simulink model "MATMPC_SIMULINK"  (R2019b)
settings: Solver=FixedStepAuto  StartTime=0.0  StopTime=1  RelTol=1e-3
undefined symbols (not defined in the file or in its folder): indata, opt, settings, Ts, x0
libraries: dspindex x1
settings Model: Creator=chen  LastModifiedBy=ichelikh
settings DataIOCC: ReturnWorkspaceOutputs=off
settings DebuggingCC: ArithmeticOperatorsInVariantConditions=warning
settings SFSimCC: SimUseLocalCustomCode=off  CustomCodeUndefinedFunction=UseInterfaceOnly
settings RTWCC: RTWUseLocalCustomCode=off  CheckMdlBeforeBuild=Error

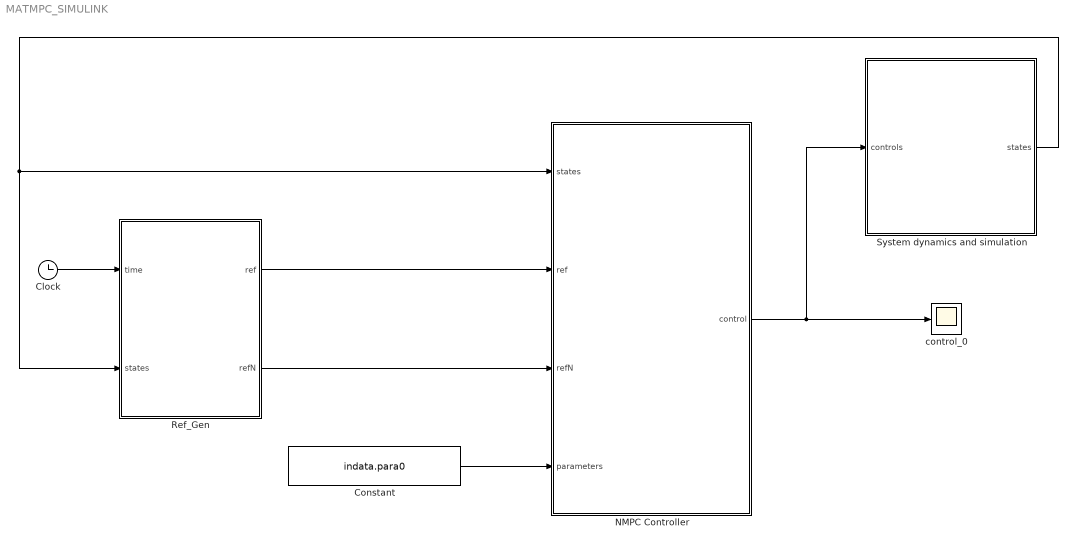
== system MATMPC_SIMULINK ==
  Clock : Clock
  Constant : Constant  Value=indata.para0
  NMPC Controller : Subsystem
  Ref_Gen : Subsystem
  System dynamics and simulation : Subsystem
  control_0 : Scope
  wires:
  NMPC Controller/1(control) -> System dynamics and simulation/1("controls "), control_0/1
  Ref_Gen/1(ref) -> NMPC Controller/2("ref ")
  Ref_Gen/2(refN) -> NMPC Controller/3("refN ")
  Constant/1 -> NMPC Controller/4(parameters)
  Clock/1 -> Ref_Gen/1(time)
  System dynamics and simulation/1(states) -> Ref_Gen/2("states "), NMPC Controller/1("states ")

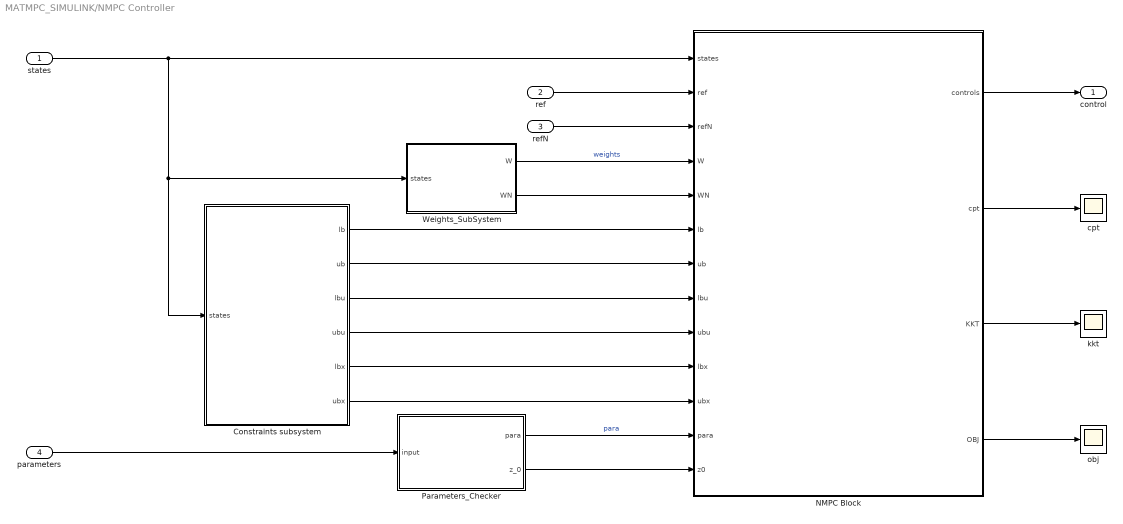
== system MATMPC_SIMULINK/NMPC Controller ==
  "states " : Inport
  "ref " : Inport  Port=2
  "refN " : Inport  Port=3
  parameters : Inport  Port=4
  Constraints subsystem : Subsystem
  "NMPC Block " : MATLAB Function  TreatAsAtomicUnit=on  SystemSampleTime=Ts
  Parameters_Checker : MATLAB Function  TreatAsAtomicUnit=on  SystemSampleTime=settings.Ts
  Weights_SubSystem : Subsystem
  cpt : Scope
  kkt : Scope
  obj : Scope
  control : Outport
  wires:
  "refN "/1 -> "NMPC Block "/3(refN)
  "NMPC Block "/4(OBJ) -> obj/1
  "NMPC Block "/3(KKT) -> kkt/1
  "NMPC Block "/2(cpt) -> cpt/1
  "ref "/1 -> "NMPC Block "/2(ref)
  "NMPC Block "/1(controls) -> control/1
  "states "/1 -> Constraints subsystem/1(states), Weights_SubSystem/1(states), "NMPC Block "/1(states)
  Weights_SubSystem/2(WN) -> "NMPC Block "/5(WN)
  Weights_SubSystem/1(W) -> "NMPC Block "/4(W)  "weights"
  Constraints subsystem/1(lb) -> "NMPC Block "/6(lb)
  Constraints subsystem/2(ub) -> "NMPC Block "/7(ub)
  Constraints subsystem/3(lbu) -> "NMPC Block "/8(lbu)
  Constraints subsystem/4(ubu) -> "NMPC Block "/9(ubu)
  Constraints subsystem/5(lbx) -> "NMPC Block "/10(lbx)
  Constraints subsystem/6(ubx) -> "NMPC Block "/11(ubx)
  Parameters_Checker/1(para) -> "NMPC Block "/12(para)  "para"
  parameters/1 -> Parameters_Checker/1(input)
  Parameters_Checker/2(z_0) -> "NMPC Block "/13(z0)

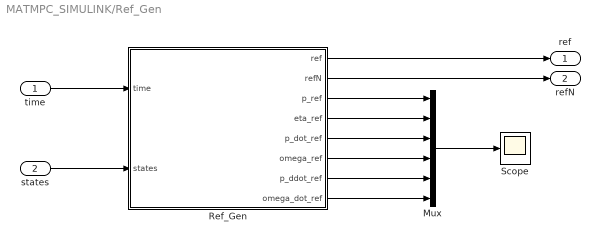
== system MATMPC_SIMULINK/Ref_Gen ==
  time : Inport
  "states " : Inport  Port=2
  Mux : Mux  Inputs=6
  Ref_Gen : MATLAB Function  TreatAsAtomicUnit=on
  Scope : Scope
  ref : Outport
  refN : Outport  Port=2
  wires:
  Ref_Gen/4(eta_ref) -> Mux/2
  Ref_Gen/3(p_ref) -> Mux/1
  Ref_Gen/8(omega_dot_ref) -> Mux/6
  Ref_Gen/2(refN) -> refN/1
  time/1 -> Ref_Gen/1(time)
  Ref_Gen/7(p_ddot_ref) -> Mux/5
  Ref_Gen/1(ref) -> ref/1
  Ref_Gen/5(p_dot_ref) -> Mux/3
  Ref_Gen/6(omega_ref) -> Mux/4
  Mux/1 -> Scope/1
  "states "/1 -> Ref_Gen/2(states)

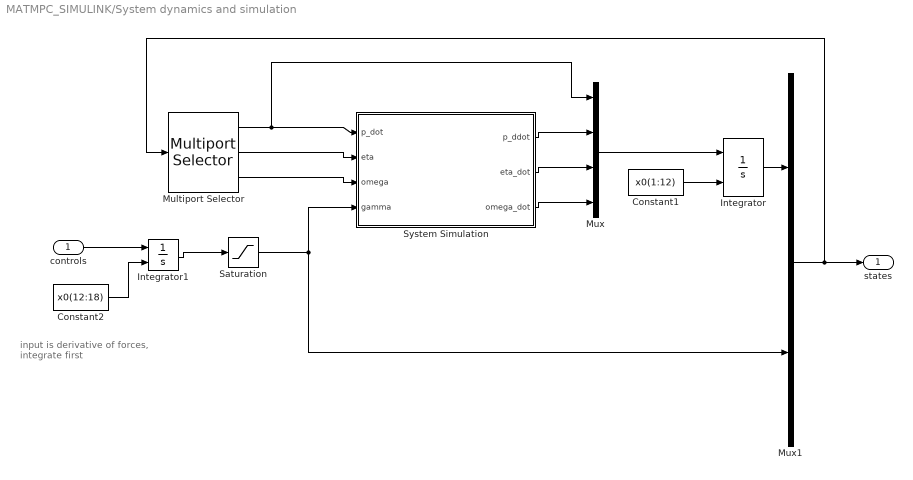
== system MATMPC_SIMULINK/System dynamics and simulation ==
  note: input is derivative of forces, integrate first
  "controls " : Inport
  Constant1 : Constant  Value=x0(1:12)
  Constant2 : Constant  Value=x0(12:18)
  Integrator : Integrator  InitialConditionSource=external  InitialCondition=x0
  Integrator1 : Integrator  InitialConditionSource=external
  Multiport Selector : dspindex/Multiport Selector  rowsOrCols=Rows  idxCellArray={ 4:6, 7:9, 10:12}  idxErrMode=Clip Index
  Mux : Mux
  Mux1 : Mux  Inputs=2
  Saturation : Saturate  UpperLimit=indata.constraints.f_max  LowerLimit=indata.constraints.f_min
  System Simulation : MATLAB Function  TreatAsAtomicUnit=on
  states : Outport
  wires:
  Integrator1/1 -> Saturation/1
  "controls "/1 -> Integrator1/1
  Saturation/1 -> Mux1/2, System Simulation/4(gamma)
  Multiport Selector/2 -> System Simulation/2(eta)
  Multiport Selector/3 -> System Simulation/3(omega)
  Constant1/1 -> Integrator/2
  Multiport Selector/1 -> Mux/1, System Simulation/1(p_dot)
  System Simulation/1(p_ddot) -> Mux/2
  System Simulation/2(eta_dot) -> Mux/3
  System Simulation/3(omega_dot) -> Mux/4
  Mux/1 -> Integrator/1
  Integrator/1 -> Mux1/1
  Mux1/1 -> states/1, Multiport Selector/1
  Constant2/1 -> Integrator1/2

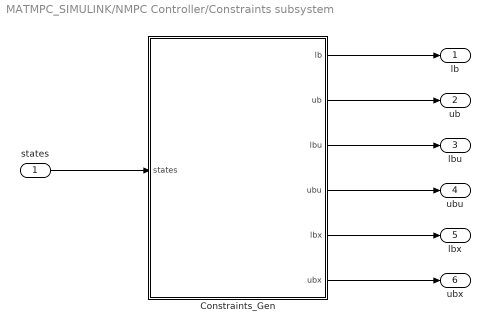
== system MATMPC_SIMULINK/NMPC Controller/Constraints subsystem ==
  states : Inport
  Constraints_Gen : MATLAB Function  TreatAsAtomicUnit=on  SystemSampleTime=settings.Ts
  lb : Outport  VectorParamsAs1DForOutWhenUnconnected=off
  ub : Outport  Port=2  VectorParamsAs1DForOutWhenUnconnected=off
  lbu : Outport  Port=3  VectorParamsAs1DForOutWhenUnconnected=off
  ubu : Outport  Port=4  VectorParamsAs1DForOutWhenUnconnected=off
  lbx : Outport  Port=5  VectorParamsAs1DForOutWhenUnconnected=off
  ubx : Outport  Port=6  VectorParamsAs1DForOutWhenUnconnected=off
  wires:
  states/1 -> Constraints_Gen/1(states)
  Constraints_Gen/5(lbx) -> lbx/1
  Constraints_Gen/3(lbu) -> lbu/1
  Constraints_Gen/6(ubx) -> ubx/1
  Constraints_Gen/1(lb) -> lb/1
  Constraints_Gen/2(ub) -> ub/1
  Constraints_Gen/4(ubu) -> ubu/1

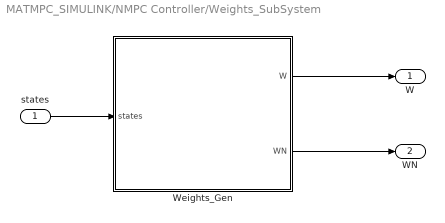
== system MATMPC_SIMULINK/NMPC Controller/Weights_SubSystem ==
  states : Inport
  Weights_Gen : MATLAB Function  TreatAsAtomicUnit=on  SystemSampleTime=settings.Ts
  W : Outport  VectorParamsAs1DForOutWhenUnconnected=off
  WN : Outport  Port=2
  wires:
  Weights_Gen/1(W) -> W/1
  states/1 -> Weights_Gen/1(states)
  Weights_Gen/2(WN) -> WN/1

== matlab function MATMPC_SIMULINK/System dynamics and simulation/System Simulation ==
  data: p_dot input size=3; eta input size=3; omega input size=3; gamma input size=nu; p_ddot output size=3; eta_dot output size=3; omega_dot output size=3; indata parameter
function [p_ddot,eta_dot,omega_dot] = Dynamic_System(p_dot, eta, omega, gamma, indata)

%% motion dynamics parameters definition
J = indata.model.J;
m = indata.model.m;
% Gravity [m/s^2]
% p     = [x; y; z];  Not needed: kept for consistency
% p_dot = [u, v, w];  Not needed: kept for consistency
% eta   = [phi; theta; psi];
% omega = eta_dot = [p; q; r];
% gamma = f = [f1; f2; f3; f4; f5; f6];

%% Extract variables

% ... from eta vector: needed to compute matrices R and T
phi = eta(1);
theta = eta(2);
psi = eta(3);

%% Initialize
g = 9.81; % gravity vector

O3 = zeros(3); % squared zero matrix of order 3
I3 = eye(3); % identity matrix of order 3
e3 = [0; 0; 1]; % z unit vector

% Generalised mass matrix
M = [m*I3 O3;
      O3  J ];

% Allocation matrix
G = [  -0.2449    0.2673   -0.2832    0.2496    0.6017   -0.5546
        0.4993   -0.4947   -0.4691    0.4971    0.0212   -0.0038
        0.7157    0.6958    0.6572    0.6714    0.7051    0.7304
       -0.0031    0.1762    0.1769   -0.0046   -0.1827   -0.1746
       -0.2100   -0.0996    0.0945    0.2112    0.1111   -0.1077
        0.1976   -0.1857    0.1864   -0.1945    0.1894   -0.1923    ];
 
% Rotation matrix from Euler Angles
r11 = cos(theta) * cos(psi);
r21 = cos(theta) * sin(psi);
r31 = -sin(theta);
r12 = sin(phi) * sin(theta) * cos(psi) - cos(phi) * sin(psi);
r22 = sin(phi) * sin(theta) * sin(psi) + cos(phi) * cos(psi);
r32 = sin(phi) * cos(theta);
r13 = cos(phi) * sin(theta) * cos(psi) + sin(phi) * sin(psi);
r23 = cos(phi) * sin(theta) * sin(psi) - sin(phi) * cos(psi);
r33 = cos(phi) * cos(theta);
R = [[r11 r21 r31].', [r12 r22 r32].', [r13 r23 r33].'];  

% Mapping matrix from eta_dot to omega
t11 = 1; t12 = 0;         t13 = -sin(theta);
t21 = 0; t22 = cos(phi);  t23 = sin(phi)*cos(theta);
t31 = 0; t32 = -sin(phi); t33 = cos(phi)*cos(theta);
T = [t11 t12 t13; t21 t22 t23; t31 t32 t33];

%% Dynamic equation of a floating-base rigid-body system

dyn_eq = M \ ([-m*g*e3; -cross(omega, J*omega)] + [R O3; O3 I3]*G*gamma);

%% Return output
% p_dot = p_dot; % unnecessary 
p_ddot = dyn_eq(1:3);
eta_dot = T \ omega;
omega_dot = dyn_eq(4:6);

return

== matlab function MATMPC_SIMULINK/NMPC Controller/NMPC Block  ==
  settings: updateMethod=DISCRETE
  data: states input size=nx; opt parameter; ref input size=[ny N]; refN input size=nyN; controls output size=[nu 1]; cpt output size=1; KKT output; OBJ output; W input; WN input; lb input; ub input; lbu input; ubu input; lbx input; ubx input; settings parameter; para input; z0 input
function [controls, cpt, KKT, OBJ] = NMPC_BLOCK(states, opt, ref, refN, W, WN, lb, ub, lbu, ubu, lbx, ubx, settings, para, z0)

%% everything should has a fixed size
coder.extrinsic('mpc_nmpcsolver_simulink');  
coder.extrinsic('InitData');  
coder.extrinsic('InitMemory');  
coder.extrinsic('evalin');
coder.extrinsic('assignin');

%%

persistent x u z lambda mu mu_x mu_u;
persistent input mem;

if isempty(input)  
    
    nx = settings.nx;        % No. of differential states
    nu = settings.nu;        % No. of controls
    nz = settings.nz;        % No. of algebraic states
    ny = settings.ny;        % No. of outputs (references)    
    nyN= settings.nyN;       % No. of outputs at terminal stage 
    np = settings.np;        % No. of parameters (on-line data)
    nc = settings.nc;        % No. of constraints
    ncN = settings.ncN;      % No. of constraints at terminal stage
    nbu = settings.nbu;      % No. of control bounds
    nbx = settings.nbx;      % No. of state bounds
    nbu_idx = settings.nbu_idx; % Index of control bounds
    nbx_idx = settings.nbx_idx; % Index of state bounds
    N = settings.N;
    N2 = settings.N2;
    r = settings.r;
        
    input.x0=states;
    
    x=repmat(states,1,N+1);
    input.x=x;
    
    u=zeros(nu,N);
    input.u=u;
    
    z=repmat(z0,1,N);
    input.z=z;
    
    lambda = zeros(nx,N+1);
    input.lambda= lambda;
    
    if N*nc+ncN > 0
        mu = zeros(N*nc+ncN,1);
    else
        mu = 0;
    end
    input.mu= mu;
    
    mu_u = zeros(N*nu,1);
    input.mu_u= mu_u;
    
    if N*nbx > 0
        mu_x = zeros(N*nbx,1);
    else
        mu_x = 0;
    end
    input.mu_x = mu_x;
    
    input.W=W;
    input.WN=WN;
    input.od = para;
    
    input.lb = lb;
    input.ub = ub;
    input.lbx = lbx;
    input.ubx = ubx;
    input.lbu = lbu;
    input.ubu = ubu;
      
    input.y = ref;
    input.yN = refN;
    
    mem = InitMemory(settings, opt, input);
        
else

    input.x=x; 
    input.u=u;
    input.z=z;
    input.lambda=lambda;   
    input.mu=mu;
    input.mu_x=mu_x;
    input.mu_u=mu_u;
    
end

%%
cpt = 0;
KKT = 0;
OBJ = 0;
input.x0 = states;
[input,mem,cpt,KKT,OBJ] = mpc_nmpcsolver_simulink(input, settings, mem, opt);
controls = input.u(:,1);

%% shifting
switch opt.shifting
    case 'yes'
        x=[input.x(:,2:end),input.x(:,end)];  
        u=[input.u(:,2:end),input.u(:,end)]; 
        z=[input.z(:,2:end),input.z(:,end)]; 
        lambda=[input.lambda(:,2:end),input.lambda(:,end)];
        if (settings.N*settings.nc+settings.ncN) >0
            mu(1:end-settings.ncN+1)=input.mu(settings.nc+1:settings.N*settings.nc+settings.ncN,1);
            mu(settings.N*settings.nc+1:end)=input.mu(settings.N*settings.nc+settings.ncN-settings.nc+1:settings.N*settings.nc+settings.ncN,1);
        else
            mu=0;
        end
        mu_x=[input.mu_x(2:end,1);input.mu_x(end,1)];
        mu_u=[input.mu_u(2:end,1);input.mu_u(end,1)];
   case 'no'
        x=input.x;
        u=input.u;
        z=input.z;
        lambda=input.lambda;
        mu=input.mu;
        mu_x=input.mu_x;
        mu_u=input.mu_u;
end

return

== matlab function MATMPC_SIMULINK/Ref_Gen/Ref_Gen ==
  data: ref output; settings parameter; refN output; time input; states input size=nx; p_ref output; eta_ref output; p_dot_ref output; omega_ref output; p_ddot_ref output; omega_dot_ref output; indata parameter
function [ref, refN, p_ref, eta_ref, p_dot_ref, omega_ref, p_ddot_ref, omega_dot_ref] = Reference_Gen(settings, time, states, indata)

persistent j motion t_start desired_WP tau W_p_B WPs;
            
%% Import variables
% ... from struct "settings"
N = settings.N;
ny = settings.ny;
nyN = settings.nyN;
nu_v = settings.nu_v;
nu_lambda = settings.nu_lambda;
Ts_st = settings.Ts_st;

% ... from vector "data"
x0 = indata.x0;

%% Initialize vectors

curr_pos = zeros(3, 1);
ref = zeros(ny, N);
refN = zeros(nyN, 1);

REF = zeros(ny, (N + 1));

p_ref = zeros(3, 1); 
eta_ref = zeros(3, 1); 
p_dot_ref = zeros(3, 1); 
omega_ref = zeros(3, 1); 
p_ddot_ref = zeros(3, 1); 
omega_dot_ref = zeros(3, 1);

%% Take current state
curr_pos(1) = states(1); % At the beginning states is equal to x0 (see Initialization_Simulink.m)
curr_pos(2) = states(2);
curr_pos(3) = states(3); 

%% Initialize default values for reference trajectory
% Some may be overwritten in next section

% Default values for desired position
x = 0; 
y = 0; 
z = 0;
% Default values for desired linear velocity
x_dot = 0; 
y_dot = 0; 
z_dot = 0;
% Default values for desired acceleration
x_ddot = 0; 
y_ddot = 0; 
z_ddot = 0;
% Default values for desired attitude
roll = 0; 
pitch = 0;             
yaw = 0; 
% Default values for desired angular velocity
omega_x = 0; 
omega_y = 0; 
omega_z = 0;
% Default values for desired angular acceleration
omega_dot_x = 0;
omega_dot_y = 0;
omega_dot_z = 0;
    
%% Generate reference trajectory
for i = 1: N+1
        
  % ........................ Sequence of waypoints ......................
  p_t0 = indata.x0(1:3); % starting position --- p(t=t0)
  h_safe = 0; % safety-height offset
  av_speeds = indata.wps.vel; % import speeds steps
  n_wps = indata.wps.num; % import number of waypoints
  if isempty(desired_WP)
      j = 1; 
      WPs = indata.wps.pos; % load sequence of waypoints
      desired_WP = WPs(:,j); % set as desired waypoint the current one
      % initialize body position in World frame (where drone 
      % should be at current time t)
      W_p_B = p_t0 + [0; 0; h_safe]; 
      t_start = indata.wps.t_start; % import time instant in which motion should start
      tau = 1;
      motion = 0;
  end
  if (time > t_start) && ~motion && j < n_wps
      desired_WP = WPs(:, j+1); % set as desired waypoint the next one
      distances = sqrt((desired_WP - WPs(:,j)).^2); % compute distance to next waypoint
      % compute time needed to reach next waypoint using 
      % corresponding constant speed step
      tau = norm(distances)/ 4.5 / av_speeds(j); 
      if tau > 0.001 % if next waypoint if far enough
          motion = 1; % trigger motion
      end
  end
  if motion % if motion has been triggered
      t = (time - t_start) / tau;
      % compute position where drone should be at current time t,
      % through a 2nd-order system response to motion step
      W_p_B = WPs(:,j) + (desired_WP - WPs(:,j)) .* (1 - exp(-t) - t*exp(-t)); 
      if norm(W_p_B - desired_WP) < 0.01 % if next waypoint has been reached
          disp('drone waypoint reached');
          disp(j+1);
          j = j+1; % point to next waypoint
          motion = 0; % reset motion trigger
          t_start = time + indata.wps.t_rest; % wait rest time before start next motion step
      end
  end
  % set as desired coordinates the position where drone should be
  % at current time t
  x = W_p_B(1); 
  y = W_p_B(2);
  z = W_p_B(3);
  % set desired yaw
  yaw = x0(9);


% Return desired reference trajectory of first shooting point for
% plotting purposes
if i == 1
    p_ref = [x y z]';
    p_dot_ref = [x_dot y_dot z_dot]';
    p_ddot_ref = [x_ddot y_ddot z_ddot]';

    eta_ref = [roll pitch yaw]';
    omega_ref = [omega_x omega_y omega_z]';
    omega_dot_ref = [omega_dot_x omega_dot_y omega_dot_z]';
end

% Reference over the time window for NMPC
REF(:, i) = [ x y z ...     % p
              roll pitch yaw ...    % eta
              x_dot y_dot z_dot ...     % p_dot
              omega_x omega_y omega_z ...   % omega
              x_ddot y_ddot z_ddot ...  % p_ddot
              omega_dot_x omega_dot_y omega_dot_z ...  % omega_dot
              0*ones(nu_v,1)' ...   % alpha_dot
              0*ones(nu_lambda,1)']'; %lambda_dot

end

%% Return output
ref = REF(:, 1:N);
refN = REF(1:end-nu_v-nu_lambda, N+1);

== matlab function MATMPC_SIMULINK/NMPC Controller/Constraints subsystem/Constraints_Gen ==
  settings: sampleTime=sim_time_step
  data: lb output size=settings.size_b; settings parameter; indata parameter; states input size=settings.nx; ub output size=settings.size_b; lbu output size=settings.size_bu; ubu output size=settings.size_bu; lbx output size=settings.size_bx; ubx output size=settings.size_bx
function [lb, ub, lbu, ubu, lbx, ubx]  = Constraints_Gen(settings, indata, states)

%% Importing 
% ... from  parameter `settings`
nu = settings.nu;
nu_lambda = settings.nu_lambda;
nu_v = settings.nu_v;
nbu = settings.nbu;
nbu_idx = settings.nbu_idx;
N = settings.N;

% ... from parameter `data`
c_f = indata.model.c_f;
omega_bar = indata.constraints.omega_bar;
dot_omega_bar_max = indata.constraints.dot_omega_bar_max;
dot_omega_bar_min = indata.constraints.dot_omega_bar_min;
coeff_angular_acc = indata.constraints.coeff_angular_acc;
coeff_angular_dec = indata.constraints.coeff_angular_dec;
%
dot_alpha_min = indata.constraints.dot_alpha_min;
dot_alpha_max = indata.constraints.dot_alpha_max;

% ... from input `states`
% State-dependent constraints
F = zeros(0,1);
for k = 0:nu-1
    F = [F;states(13+k)];
end
% f1 = states(13);
% f2 = states(14);
% f3 = states(15);
% f4 = states(16);
% f5 = states(17);
% f6 = states(18);

%% Variables definition

% vector F
% F = [f1; f2; f3; f4; f5; f6];

% Define the bounds of Delta U from equation:
%   dot_f(t) = 2 * kf * omega_i(t) * dot_omega_i(t),
%   where i is the i-th propeller 

%% Upper and lower bounds for general constraints 
% Dimensions of lb_g and ub_g should be equal to nc.
lb_g = [];
ub_g = [];

% Dimensions of lb_gN and ub_gN should be equal to ncN.
lb_gN = [];
ub_gN = [];

lb_g_rep = repmat(lb_g, N, 1);
ub_g_rep = repmat(ub_g, N, 1);

lb_temp = [lb_g_rep; lb_gN];
ub_temp = [ub_g_rep; ub_gN];

if isempty(lb_temp | ub_temp)
    
    lb = 0;
    ub = 0;

else
    
    lb = lb_temp;
    ub = ub_temp;
    
end

%% Lower and upper bounds for input 
% Dimensions of lb_u and ub_u should be equal to nbu.
lb_u = zeros(nbu, 1);
ub_u = zeros(nbu, 1);

% Propeller upper and lower bounds computation
% The bounds depend on current state of TiltHex. 
% This computation is repeated for each propeller
dot_omega_temp_acc = zeros(nu_lambda, 1);
dot_omega_temp_dec = zeros(nu_lambda, 1);

for i = 1:nu_lambda
% At each value inside omega_bar corresponds an upper and lower bound of dot_omega_bar,
% taken rispectively inside dot_omega_bar_max and dot_omega_bar_min.
% First it is mandatory to understand in which interval is the force provided
% by the i-th propeller; omega_bar values are translated into force
% quantities by F = k_f*omega^2 relationship, then i-th propeller's force is 
% compared to those value in order to understand in which interval the i-th 
% propeller is working. Then, once found the interval, linear interpolation 
% is used to adjust upper and lower bounds of extremity points of that
% interval to the actual in-between point.
        
        % If less force is requested w.r.t. the first upper and lower
        % bounds, then use first elements of omega_bar_min and _max
        % AND ALSO (update Davide & Youssef 01/06/2021) set the lower and
        % upper limits for the input equal to the same limits of the first
        % (smaller) spinning velocity setpoint. 
        % This is done to avoid the if a propeller is spinnijg with zero
        % velocity also his bounds of acceleration are set to zero; we
        % don't want this. Therefore, a minimum acceleration/deceleration
        % is always guaranteed.
        f_first_setpoint = c_f(i) * omega_bar(1)^2;
        if (abs(F(i)) <= f_first_setpoint)
            dot_omega_temp_acc(i) = dot_omega_bar_max(1);
            dot_omega_temp_dec(i) = dot_omega_bar_min(1);
            ub_u(i) = 2 * sqrt(f_first_setpoint * c_f(i)) * dot_omega_bar_max(1);
            lb_u(i) = 2 * sqrt(f_first_setpoint * c_f(i)) * dot_omega_bar_min(1);
        
        % Otherwise you need to interpolate, depending at which omega the
        % i-th propeller is spinning. 
        elseif (abs(F(i)) > c_f(i) * omega_bar(1)^2 && abs(F(i)) <= c_f(i) * omega_bar(2)^2)
            dot_omega_temp_acc(i) = (coeff_angular_acc(1) * (sqrt(abs(F(i)) / c_f(i)) - omega_bar(2)) + dot_omega_bar_max(2));
            dot_omega_temp_dec(i) = (coeff_angular_dec(1) * (sqrt(abs(F(i)) / c_f(i)) - omega_bar(2)) + dot_omega_bar_min(2));
            ub_u(i)= 2 * sqrt(abs(F(i)) * c_f(i)) * dot_omega_temp_acc(i);
            lb_u(i)= 2 * sqrt(abs(F(i)) * c_f(i)) * dot_omega_temp_dec(i);
            
        elseif (abs(F(i)) > c_f(i) * omega_bar(2)^2 && abs(F(i)) <= c_f(i) * omega_bar(3)^2)
            dot_omega_temp_acc(i) = (coeff_angular_acc(2) * (sqrt(abs(F(i)) / c_f(i)) - omega_bar(3)) + dot_omega_bar_max(3));
            dot_omega_temp_dec(i) = (coeff_angular_dec(2) * (sqrt(abs(F(i)) / c_f(i)) - omega_bar(3)) + dot_omega_bar_min(3));
            ub_u(i) = 2 * sqrt(abs(F(i)) * c_f(i)) * dot_omega_temp_acc(i);
            lb_u(i) = 2 * sqrt(abs(F(i)) * c_f(i)) * dot_omega_temp_dec(i);
        
        elseif (abs(F(i)) > c_f(i) * omega_bar(3)^2 && abs(F(i)) <= c_f(i) * omega_bar(4)^2)
            dot_omega_temp_acc(i) = (coeff_angular_acc(3) * (sqrt(abs(F(i)) / c_f(i)) - omega_bar(4)) + dot_omega_bar_max(4));
            dot_omega_temp_dec(i) = (coeff_angular_dec(3) * (sqrt(abs(F(i)) / c_f(i)) - omega_bar(4)) + dot_omega_bar_min(4));
            ub_u(i) = 2 * sqrt(abs(F(i)) * c_f(i)) * dot_omega_temp_acc(i);
            lb_u(i) = 2 * sqrt(abs(F(i)) * c_f(i)) * dot_omega_temp_dec(i);
        
        elseif (abs(F(i)) > c_f(i) * omega_bar(4)^2 && abs(F(i)) <= c_f(i) * omega_bar(5)^2)
            dot_omega_temp_acc(i) = (coeff_angular_acc(4) * (sqrt(abs(F(i)) / c_f(i)) - omega_bar(5)) + dot_omega_bar_max(5));
            dot_omega_temp_dec(i) = (coeff_angular_dec(4) * (sqrt(abs(F(i)) / c_f(i)) - omega_bar(5)) + dot_omega_bar_min(5));
            ub_u(i)= 2 * sqrt(abs(F(i)) * c_f(i)) * dot_omega_temp_acc(i);
            lb_u(i)= 2 * sqrt(abs(F(i)) * c_f(i)) * dot_omega_temp_dec(i);
        
        elseif (abs(F(i)) > c_f(i) * omega_bar(5)^2 && abs(F(i)) <= c_f(i) * omega_bar(6)^2)
            dot_omega_temp_acc(i) = (coeff_angular_acc(5) * (sqrt(abs(F(i)) / c_f(i)) - omega_bar(6)) + dot_omega_bar_max(6));
            dot_omega_temp_dec(i) = (coeff_angular_dec(5) * (sqrt(abs(F(i)) / c_f(i)) - omega_bar(6)) + dot_omega_bar_min(6));
            ub_u(i) = 2 * sqrt(abs(F(i)) * c_f(i)) * dot_omega_temp_acc(i);
            lb_u(i) = 2 * sqrt(abs(F(i)) * c_f(i)) * dot_omega_temp_dec(i);
        
        elseif (abs(F(i)) > c_f(i) * omega_bar(6)^2)
            dot_omega_temp_acc(i) = (coeff_angular_acc(6) * (sqrt(abs(F(i)) / c_f(i)) - omega_bar(7)) + dot_omega_bar_max(7));
            dot_omega_temp_dec(i) = (coeff_angular_dec(6) * (sqrt(abs(F(i)) / c_f(i)) - omega_bar(7)) + dot_omega_bar_min(7));
            ub_u(i) = 2 * sqrt(abs(F(i)) * c_f(i)) * dot_omega_temp_acc(i);
            lb_u(i) = 2 * sqrt(abs(F(i)) * c_f(i)) * dot_omega_temp_dec(i);
        end
end

%
for i = nu_lambda+1:nu_lambda+nu_v
    ub_u(i) = dot_alpha_max;
    lb_u(i) = dot_alpha_min;   
end
%

lbu_temp = -inf(nu, 1);
ubu_temp = inf(nu, 1);

for i = 1:nbu
    lbu_temp(nbu_idx(i)) = lb_u(i);
    ubu_temp(nbu_idx(i)) = ub_u(i);
end

lbu = repmat(lbu_temp, 1, N);
ubu = repmat(ubu_temp, 1, N);

%% Lower and upper bounds for state 
lb_x = indata.constraints.lbx;
ub_x = indata.constraints.ubx;

if isempty(lb_x | ub_x)    
    lbx = zeros(1, N);
    ubx = zeros(1, N);
else
    lbx = repmat(lb_x, 1, N);
    ubx = repmat(ub_x, 1, N);
end

end

== matlab function MATMPC_SIMULINK/NMPC Controller/Parameters_Checker ==
  data: para output size=settings.size_od; settings parameter; input input; z_0 output
function [para, z_0]  = Parameters_Checker(settings, input)
% PARA_GENERATOR Prepares para matrix for NMPC solver. 
%
% Para is a matrix containing all the params values over all shooting
% points. Each column j is a vector containing params values for the j-th
% shooting point. Therefore the para matrix must have the number of rows
% equal to the number of params and number of columns equal to N+1, where N
% is the number of shooting points.
%
%   para PARA_GENERATOR(input, settings)
%     
%     Inputs:
%     ---------------------------------------------------------------------
%       - input: struct containing all params. Each field is a different
%                param
%
%       - settings: struct containing data related to the settings used in
%                   the simulation
%           -> Ts: sampling time [s] (i.e. time at which the controller
%                  works)
%           -> Ts_st: shooting interval [s], i.e. temporal distance between 
%                     one shooting point and the next one
%           -> s: number of integration steps per interval
%           -> nx: no. of states
%           -> nu: no. of controls
%           -> ny: no. of outputs (references)    
%           -> nyN: no. of outputs at terminal stage 
%           -> np: no. of parameters (on-line data)
%           -> nc: no. of constraints
%           -> ncN: no. of constraints at terminal stage
%           -> nbu: no. of control bounds
%           -> nbx: no. of state bounds
%           -> nbu_idx: index of control bounds
%           -> nbx_idx: index of state bounds
%           -> N: no. of shooting points
%           -> N2: no. of partial condensing blocks 
%           -> r: no. of input move blocks
%
%     Outputs:
%     ---------------------------------------------------------------------
%       - para: matrix containing all the params values over all shooting
%               points. Each column j is a vector containing params values 
%               for the j-th shooting point. Its dimension is
%               [no_of_params, N+1], where N is the number of shooting
%               points

    %% Extracting variables from settings struct
    
    % Number of shooting points
    N = settings.N;
    np = settings.np;
    nz = settings.nz;
    %% Arraging params in para vector
    % para must be a matrix, where each column j is the vector of params of
    % the j-th shooting point
    
    if np > 0
        input_rows = size(input, 1);
        input_columns = size(input, 2);
        if input_rows == np && input_columns == N+1
            para = input;
        else
            error('NMPC para vector has invalid size!');
        end
    else
        para = zeros(1, N+1); % see settings.size_od
    end
    z_0 = settings.z0;
     % faire un bloc espace algebrique 
    % Sice at the beginning of the NMPC solver this param is constant over
    % all shooting points, replicate it over n+1 column
%     para = repmat(params, 1, N+1); % dimension = [n_of_params, N+1], where N is the number of shooting points
end

== matlab function MATMPC_SIMULINK/NMPC Controller/Weights_SubSystem/Weights_Gen ==
  settings: sampleTime=sim_time_step
  data: W output size=settings.size_W; settings parameter; indata parameter; states input size=settings.nx; WN output size=settings.size_WN
function [W, WN]  = Weights_Gen(settings, indata, states)
%% Importing variables 
% ... from parameter `settings`
nyN = settings.nyN;
N = settings.N;

% ... from parameter `data`
q = indata.weights.q;

% ... from input `states`

%% Do something here

%% Format correctly weights for the cost function
W = repmat(q', 1, N);
WN = W(1:nyN, 1);
